simulink model "CA3_model"  (R2021a)
settings: Solver=VariableStepAuto  StartTime=0.0  StopTime=300  RelTol=1e-3
values from neighbouring files (symbols this model uses):
  b = [0;1]    [CA3.m]
  C = 0.5    [CA3.m]
  Gamma = [ 1 0 ... (first row only)    [CA3.m]
  gamma = 100    [CA3.m]
  K = 6.2    [CA3.m]
  P = lyap(Am',Q)    [CA3.m]
  tau = 0.25    [CA3.m]
  w = 10    [CA3.m]
undefined symbols (not defined in the file or in its folder): variance
settings Model: Creator=Administrator  LastModifiedBy=Administrator

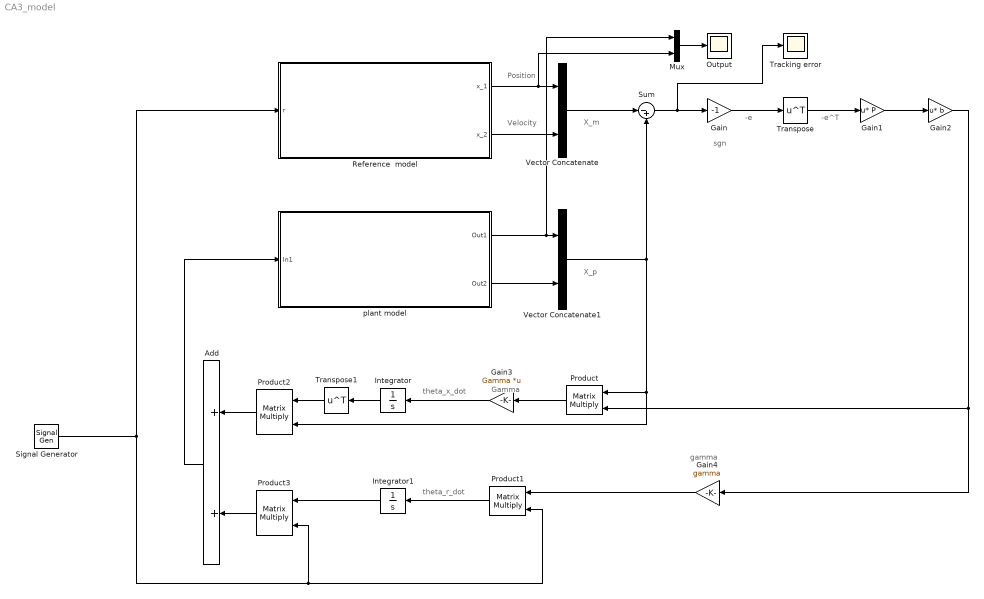
== system CA3_model ==
  note: -e^T
  note: sgn
  note: -e
  note: Gamma
  note: gamma
  note: Position
  note: Velocity
  note: X_m
  note: X_p
  note: theta_x_dot
  note: theta_r_dot
  Add : Sum
  Gain : Gain  Gain=-1
  Gain1 : Gain  Gain=P  Multiplication=Matrix(u*K)
  Gain2 : Gain  Gain=b  Multiplication=Matrix(u*K)
  Gain3 : Gain  Gain=Gamma  Multiplication=Matrix(K*u)
  Gain4 : Gain  Gain=gamma
  Integrator : Integrator
  Integrator1 : Integrator
  Mux : Mux  Inputs=2
  Output : Scope
  Product{,1..3} (4 alike) : Product  Multiplication=Matrix(*)
  Reference  model : Subsystem
  Signal Generator : SignalGenerator  WaveForm=square  Frequency=0.05
  Sum : Sum  Inputs=|-+
  Tracking error : Scope
  Transpose : Math  Operator=transpose  SaturateOnIntegerOverflow=on
  Transpose1 : Math  Operator=transpose  SaturateOnIntegerOverflow=on
  Vector Concatenate : Concatenate  Mode=Multidimensional array
  Vector Concatenate1 : Concatenate  Mode=Multidimensional array
  plant model : Subsystem
  wires:
  Gain/1 -> Transpose/1
  Transpose/1 -> Gain1/1
  Gain1/1 -> Gain2/1
  Gain2/1 -> Product/2, Gain4/1
  Reference  model/1(x_1) -> Mux/2, Vector Concatenate/1
  Reference  model/2(x_2) -> Vector Concatenate/2
  Vector Concatenate1/1 -> Product/1, Product2/2, Sum/2
  Gain4/1 -> Product1/1
  Integrator/1 -> Transpose1/1
  Transpose1/1 -> Product2/1
  Product1/1 -> Integrator1/1
  Integrator1/1 -> Product3/1
  Product2/1 -> Add/1
  Signal Generator/1 -> Reference  model/1(r), Product1/2, Product3/2
  Sum/1 -> Tracking error/1, Gain/1
  Vector Concatenate/1 -> Sum/1
  Product/1 -> Gain3/1
  Gain3/1 -> Integrator/1
  plant model/1(Out1) -> Mux/1, Vector Concatenate1/1
  plant model/2(Out2) -> Vector Concatenate1/2
  Product3/1 -> Add/2
  Add/1 -> plant model/1(In1)
  Mux/1 -> Output/1

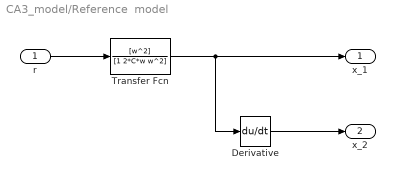
== system CA3_model/Reference  model ==
  r : Inport
  Derivative : Derivative
  Transfer Fcn : TransferFcn  Numerator=[w^2]  Denominator=[1 2*C*w w^2]
  x_1 : Outport
  x_2 : Outport  Port=2
  wires:
  r/1 -> Transfer Fcn/1
  Transfer Fcn/1 -> Derivative/1, x_1/1
  Derivative/1 -> x_2/1

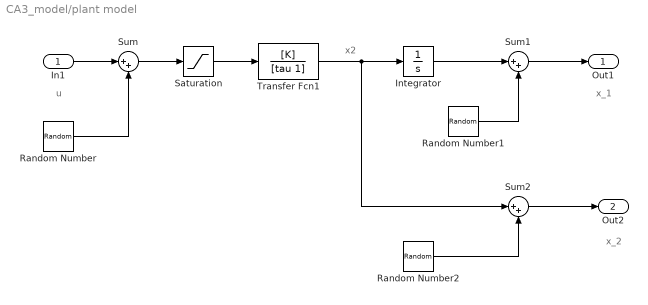
== system CA3_model/plant model ==
  note: u
  note: x_2
  note: x_1
  note: x2
  In1 : Inport
  Integrator : Integrator
  Random Number : RandomNumber  Variance=variance  SampleTime=0.1
  Random Number1 : RandomNumber  Variance=variance  SampleTime=0.1
  Random Number2 : RandomNumber  Variance=variance  SampleTime=0.1
  Saturation : Saturate  UpperLimit=5  LowerLimit=-5
  Sum : Sum  Inputs=|++
  Sum1 : Sum  Inputs=|++
  Sum2 : Sum  Inputs=|++
  Transfer Fcn1 : TransferFcn  Numerator=[K]  Denominator=[tau 1]
  Out1 : Outport
  Out2 : Outport  Port=2
  wires:
  Transfer Fcn1/1 -> Sum2/1, Integrator/1
  Random Number/1 -> Sum/2
  Saturation/1 -> Transfer Fcn1/1
  Sum/1 -> Saturation/1
  In1/1 -> Sum/1
  Integrator/1 -> Sum1/1
  Sum1/1 -> Out1/1
  Random Number1/1 -> Sum1/2
  Sum2/1 -> Out2/1
  Random Number2/1 -> Sum2/2
